simulink model "controller_dual"  (R2023a)
settings: Solver=FixedStepDiscrete  StartTime=0.0  StopTime=1.0  FixedStep=Ts  RelTol=1e-3
undefined symbols (not defined in the file): i_ref_max, K_i_i_norm, K_i_omega, K_p_i_norm, K_p_omega, Kaw_i, Kaw_w, Ts
settings Model: Creator=StarkJia  LastModifiedBy=StarkJia
settings DataIOCC: SaveFormat=StructureWithTime

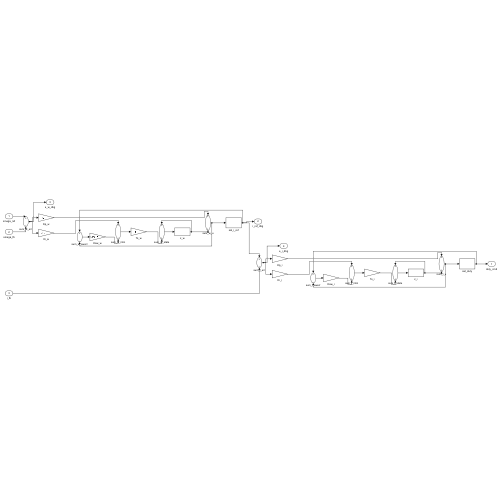
[thumbnail: Simulink's stored preview of the top-level diagram]
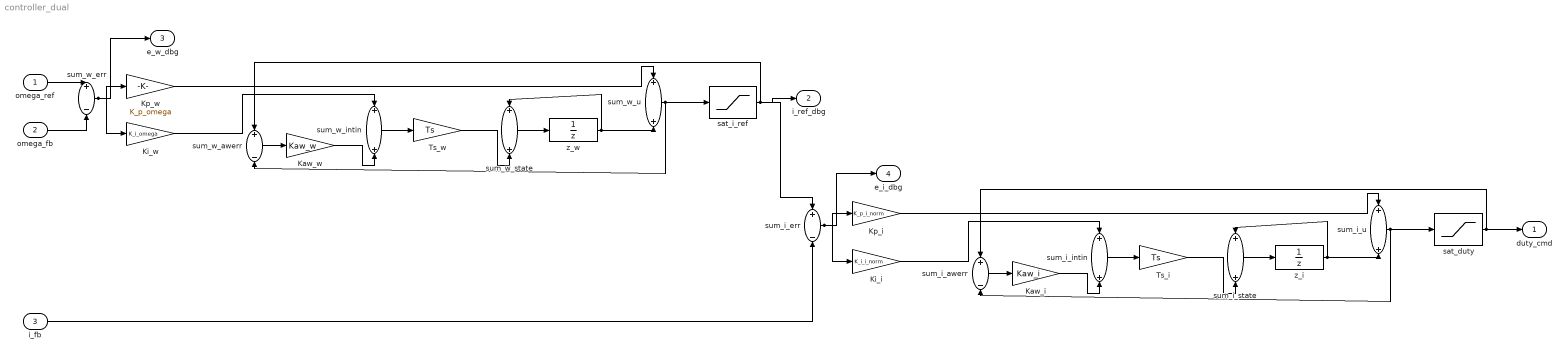
== system controller_dual ==
  omega_ref : Inport
  omega_fb : Inport  Port=2
  i_fb : Inport  Port=3
  Kaw_i : Gain  Gain=Kaw_i
  Kaw_w : Gain  Gain=Kaw_w
  Ki_i : Gain  Gain=K_i_i_norm
  Ki_w : Gain  Gain=K_i_omega
  Kp_i : Gain  Gain=K_p_i_norm
  Kp_w : Gain  Gain=K_p_omega
  Ts_i : Gain  Gain=Ts
  Ts_w : Gain  Gain=Ts
  sat_duty : Saturate  UpperLimit=1  LowerLimit=-1
  sat_i_ref : Saturate  UpperLimit=i_ref_max  LowerLimit=-i_ref_max
  sum_i_awerr : Sum  Inputs=+-
  sum_i_err : Sum  Inputs=+-
  sum_i_intin : Sum
  sum_i_state : Sum
  sum_i_u : Sum
  sum_w_awerr : Sum  Inputs=+-
  sum_w_err : Sum  Inputs=+-
  sum_w_intin : Sum
  sum_w_state : Sum
  sum_w_u : Sum
  z_i : UnitDelay  SampleTime=Ts  HasFrameUpgradeWarning=on
  z_w : UnitDelay  SampleTime=Ts  HasFrameUpgradeWarning=on
  duty_cmd : Outport
  i_ref_dbg : Outport  Port=2
  e_w_dbg : Outport  Port=3
  e_i_dbg : Outport  Port=4
  wires:
  omega_ref/1 -> sum_w_err/1
  omega_fb/1 -> sum_w_err/2
  sum_w_err/1 -> Kp_w/1, Ki_w/1, e_w_dbg/1
  Ki_w/1 -> sum_w_intin/1
  sum_w_awerr/1 -> Kaw_w/1
  Kaw_w/1 -> sum_w_intin/2
  sum_w_intin/1 -> Ts_w/1
  Ts_w/1 -> sum_w_state/2
  z_w/1 -> sum_w_state/1, sum_w_u/2
  sum_w_state/1 -> z_w/1
  Kp_w/1 -> sum_w_u/1
  sum_w_u/1 -> sat_i_ref/1, sum_w_awerr/2
  sat_i_ref/1 -> sum_w_awerr/1, i_ref_dbg/1, sum_i_err/1
  i_fb/1 -> sum_i_err/2
  sum_i_err/1 -> Kp_i/1, Ki_i/1, e_i_dbg/1
  Ki_i/1 -> sum_i_intin/1
  sum_i_awerr/1 -> Kaw_i/1
  Kaw_i/1 -> sum_i_intin/2
  sum_i_intin/1 -> Ts_i/1
  Ts_i/1 -> sum_i_state/2
  z_i/1 -> sum_i_state/1, sum_i_u/2
  sum_i_state/1 -> z_i/1
  Kp_i/1 -> sum_i_u/1
  sum_i_u/1 -> sat_duty/1, sum_i_awerr/2
  sat_duty/1 -> sum_i_awerr/1, duty_cmd/1
